simulink model "lab_5_qpsk_viterbi_sqrt"  (Simulink 7.6)
settings: Solver=VariableStepDiscrete  SolverMode=SingleTasking  StartTime=0.0  StopTime=500  RelTol=1e-3
values from neighbouring files (symbols this model uses):
  EbNodB = (1/4) * Nvar + 5    [lab_5_Pber.m]    (also in lab_5_Propyskna_Zdatnist.m = 8.5; lab_5_parameters.m = 8.5)
  Rb = Nvar    (= 14)    [lab_5_Propyskna_Zdatnist.m]    (also in lab_5_parameters.m)
  Tb = 1/Rb    (= 0.0714285714286)    [lab_5_Propyskna_Zdatnist.m]    (also in lab_5_parameters.m)
undefined symbols (not defined in the file or in its folder): figposition, Fs, sided, Two
libraries: commsink2 x6, commcnvcod2 x2, commdigbbndpm2 x2, dspsnks4 x2, commchan3 x1, commrandsrc2 x1, dspsigops x1, commfilt2 x1
CloseFcn:
  | clear convSigsOut
settings Model: RequirementInfo=9  Creator=mikem  LastModifiedBy=Sergey  CovMetricSettings=d  ExtModeTrigMode=oneshot  ExtModeArmWhenConnect=off
settings DataIOCC: LimitDataPoints=off  SaveOutput=off  SaveTime=off  SignalLoggingName=convSigsOut
settings OptimizationCC: BlockReduction=off  BooleanDataType=off  InitFltsAndDblsToZero=on
settings DebuggingCC: SaveWithParameterizedLinksMsg=none  SignalResolutionControl=TryResolveAllWithWarning  SolverPrmCheckMsg=none  MultiTaskDSMMsg=warning  MultiTaskCondExecSysMsg=none  IntegerOverflowMsg=none  StrictBusMsg=None
settings HardwareCC: TargetUnknown=on
settings RTWCC: IncludeERTFirstTime=on
settings GRTTargetCC: TargetFcnLib=ansi_tfl_tmw.mat

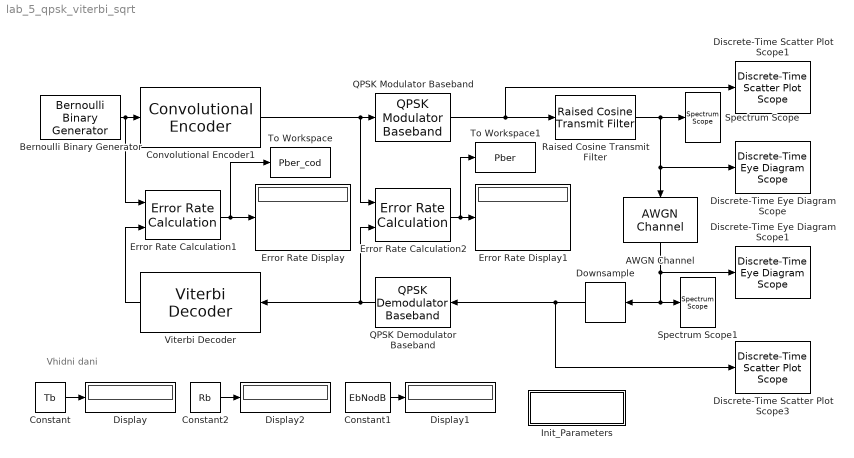
== system lab_5_qpsk_viterbi_sqrt ==
  note: Vhidni dani
  AWGN Channel : commchan3/AWGN Channel  SystemSampleTime=-1  InputProcessing=Inherited (this choice will be removed - see release notes)  seed=54321  noiseMode="Signal to noise ratio  (Es/No)"  EbNodB=5  EsNodB=EbNodB+10*log10(1/2)  SNRdB=5  bitsPerSym=2  Ps=1  Tsym=1/8*Tb  variance=1
  Bernoulli Binary Generator : commrandsrc2/Bernoulli Binary Generator  DialogController=commDDGCreate  DialogControllerArgs=DataTag1  SystemSampleTime=-1  P=0.5  seed=12345  Ts=Tb  frameBased=on  sampPerFrame=1  orient=off  outDataType=double
  Constant : Constant  Value=Tb
  Constant1 : Constant  Value=EbNodB
  Constant2 : Constant  Value=Rb
  Convolutional Encoder1 : commcnvcod2/Convolutional Encoder  trellis=poly2trellis(7, [171 133])  opMode=Continuous  DelayedResetAction=off  hasIniStPort=off  hasFinStPort=off  usePuncVector=off  punctureVector=[1; 1; 0; 1; 0; 1]  reset=Unused parameter value
  Discrete-Time Eye Diagram Scope : commsink2/Discrete-Time Eye Diagram Scope  Tag=EyeDiagram  SystemSampleTime=-1  sampPerSymb=8  offsetEye=0  symbPerTrace=2  numTraces=10  numNewFrames=1  LineStyles=-  LineColors=b  dupPoints=on  fading=on  render=on  AxisGrid=on  yMin=-1.09437970392713  yMax=1.07012752212265  inphaseLabel=In-phase Amplitude  quadratureLabel=Quadrature Amplitude  openScopeAtSimStart=on  dispDiagram=In-phase and Quadrature  FrameNumber=off  FigPos=[360 54 560 644]  figTitle=Eye Diagram  block_type_=eye  numLinesMax=8
  Discrete-Time Eye Diagram Scope1 : commsink2/Discrete-Time Eye Diagram Scope  Tag=EyeDiagram  SystemSampleTime=-1  sampPerSymb=8  offsetEye=0  symbPerTrace=2  numTraces=100  numNewFrames=1  LineStyles=-  LineColors=b  dupPoints=on  fading=on  render=on  AxisGrid=on  yMin=-1.05  yMax=1.05  inphaseLabel=In-phase Amplitude  quadratureLabel=Quadrature Amplitude  openScopeAtSimStart=on  dispDiagram=In-phase and Quadrature  FrameNumber=off  FigPos=[360 54 560 644]  figTitle=Eye Diagram  block_type_=eye  numLinesMax=8
  Discrete-Time Scatter Plot Scope1 : commsink2/Discrete-Time Scatter Plot Scope  Tag=ScatterPlot  SystemSampleTime=-1  sampPerSymb=1  offsetEye=0  numTraces=40  numNewFrames=10  LineMarkers=.  LineColors=b  fading=on  render=on  AxisGrid=on  xMin=-1.5  xMax=1.5  yMin=-1.5  yMax=1.5  inphaseLabel=In-phase Amplitude  quadratureLabel=Quadrature Amplitude  openScopeAtSimStart=on  FrameNumber=off  FigPos=[360 138 560 560]  figTitle=Scatter Plot  numLinesMax=8  block_type_=scatter
  Discrete-Time Scatter Plot Scope3 : commsink2/Discrete-Time Scatter Plot Scope  Tag=ScatterPlot  SystemSampleTime=-1  sampPerSymb=1  offsetEye=0  numTraces=40  numNewFrames=10  LineMarkers=.  LineColors=b  fading=on  render=on  AxisGrid=on  xMin=-1.5  xMax=1.5  yMin=-1.5  yMax=1.5  inphaseLabel=In-phase Amplitude  quadratureLabel=Quadrature Amplitude  openScopeAtSimStart=on  FrameNumber=off  FigPos=[360 138 560 560]  figTitle=Scatter Plot  numLinesMax=8  block_type_=scatter
  Display : Display
  Display1 : Display
  Display2 : Display
  Downsample : dspsigops/Downsample  N=8  phase=0  InputProcessing=Inherited (this choice will be removed - see release notes)  RateOptions=Enforce single-rate processing  smode=Allow multirate  fmode=Maintain input frame rate  ic=0
  Error Rate Calculation1 : commsink2/Error Rate Calculation  N=3/1*1+96  st_delay=0  cp_mode=Entire frame  subframe=[]  PMode=Port  WsName=ErrorVec  RsMode2=off  stop=off  numErr=100  maxBits=1e7
  Error Rate Calculation2 : commsink2/Error Rate Calculation  N=3/1*2  st_delay=0  cp_mode=Entire frame  subframe=[]  PMode=Port  WsName=ErrorVec  RsMode2=off  stop=off  numErr=100  maxBits=1e6
  Error Rate Display : Display
  Error Rate Display1 : Display
  Init_Parameters : Subsystem
      settings: OpenFcn=lab_5_parameters
      mask Display: disp('lab_5_parameters')
  QPSK Demodulator Baseband : commdigbbndpm2/QPSK Demodulator Baseband  SystemSampleTime=-1  OutType=Bit  Dec=Gray  Ph=pi/4  numSamp=1
  QPSK Modulator Baseband : commdigbbndpm2/QPSK Modulator Baseband  SystemSampleTime=-1  InType=Bit  Enc=Gray  Ph=pi/4  numSamp=1
  Raised Cosine Transmit Filter : commfilt2/Raised Cosine Transmit Filter  DialogController=dspDDGCreate  DialogControllerArgs=DataTag4  SystemSampleTime=-1  filtType=Normal  D=3  R=0.5  sampMode=Mute  saveAsFlag=0  N=8  framing=Maintain input frame rate  InputProcessing=Columns as channels (frame based)  checkGain=Normalized  filterGain=1  checkCoeff=off  variableName=rcTxFilt  launchFVT=off  roundingMode=Floor  overflowMode=off
      link override Check Signal Attributes: Frame=Frame-based  Dimensions=Column vector (2-D) or scalar
      link override FIR Interpolation: framing=Maintain input frame rate
  Spectrum Scope : dspsnks4/Spectrum Scope  DialogController=dspdialog.SpectrumScope  DialogControllerArgs=DataTag5  SystemSampleTime=-1  ScopeProperties=on  Domain=Frequency  HorizSpan=1  UseBuffer=on  BufferSize=256  Overlap=0  inpFftLenInherit=off  FFTlength=128  numAvg=20  DisplayProperties=off  AxisGrid=on  Memory=off  FrameNumber=off  AxisLegend=off  AxisZoom=off  OpenScopeAtSimStart=on  OpenScopeImmediately=off  FigPos="figposition([7    12    39    27])"  AxisProperties=off  XUnits=Hertz  XRange=Two-sided ((-Fs/2...Fs/2])  XDisplay=0  InheritXIncr=on  XIncr=1.0  XLabel=Samples  XLimit=Auto  YUnits=dBW/Hertz  XMax=1  XMin=0  YLabel=Magnitude-squared, dB  LineProperties=off  LineColors=[1 0 0]  wintypeSpecScope=Hann  RsSpecScope=50  betaSpecScope=5  winsampSpecScope=Periodic  XAxisParamsVer=6.8
      settings: YMin=-80  YMax=10
  Spectrum Scope1 : dspsnks4/Spectrum Scope  DialogController=dspdialog.SpectrumScope  DialogControllerArgs=DataTag6  SystemSampleTime=-1  ScopeProperties=on  Domain=Frequency  HorizSpan=1  UseBuffer=on  BufferSize=256  Overlap=0  inpFftLenInherit=off  FFTlength=128  numAvg=20  DisplayProperties=off  AxisGrid=on  Memory=off  FrameNumber=off  AxisLegend=off  AxisZoom=off  OpenScopeAtSimStart=on  OpenScopeImmediately=off  FigPos="figposition([49    12    39    27])"  AxisProperties=off  XUnits=Hertz  XRange=Two-sided ((-Fs/2...Fs/2])  XDisplay=0  InheritXIncr=on  XIncr=1.0  XLabel=Samples  XLimit=Auto  YUnits=dBW/Hertz  XMax=1  XMin=0  YLabel=Magnitude-squared, dB  LineProperties=off  LineColors=[1 0 0]  wintypeSpecScope=Hann  RsSpecScope=50  betaSpecScope=5  winsampSpecScope=Periodic  XAxisParamsVer=6.8
      settings: YMin=-50  YMax=10
  To Workspace : ToWorkspace  VariableName=Pber_cod  SampleTime=-1  SaveFormat=Array
      settings: MaxDataPoints=1
  To Workspace1 : ToWorkspace  VariableName=Pber  SampleTime=-1  SaveFormat=Array
      settings: MaxDataPoints=1
  Viterbi Decoder : commcnvcod2/Viterbi Decoder  DialogController=commDDGCreate  DialogControllerArgs=DataTag7  trellis=poly2trellis(7, [171 133])  isPunctured=off  punctureVector=[1; 1; 0; 1; 0; 1]  erasures=off  dectype=Hard decision  runSigValErrCheck=off  nsdecb=4  smWordLength=16  tbdepth=96  opmode=Continuous  reset=off  outDataType=double
  wires:
  Convolutional Encoder1/1 -> QPSK Modulator Baseband/1, Error Rate Calculation2/1
  Viterbi Decoder/1 -> Error Rate Calculation1/2
  QPSK Modulator Baseband/1 -> Raised Cosine Transmit Filter/1, Discrete-Time Scatter Plot Scope1/1
  Raised Cosine Transmit Filter/1 -> AWGN Channel/1, Discrete-Time Eye Diagram Scope/1, Spectrum Scope/1
  QPSK Demodulator Baseband/1 -> Viterbi Decoder/1, Error Rate Calculation2/2
  Bernoulli Binary Generator/1 -> Convolutional Encoder1/1, Error Rate Calculation1/1
  AWGN Channel/1 -> Downsample/1, Spectrum Scope1/1, Discrete-Time Eye Diagram Scope1/1
  Downsample/1 -> Discrete-Time Scatter Plot Scope3/1, QPSK Demodulator Baseband/1
  Error Rate Calculation1/1 -> Error Rate Display/1, To Workspace/1
  Error Rate Calculation2/1 -> Error Rate Display1/1, To Workspace1/1
  Constant/1 -> Display/1
  Constant1/1 -> Display1/1
  Constant2/1 -> Display2/1

== system lab_5_qpsk_viterbi_sqrt/Init_Parameters ==
